simulink model "question3Sim"  (R2014a)
settings: Solver=ode45  StartTime=0.0  StopTime=2  RelTol=1e-3
settings Model: Creator=cunnia3  LastModifiedBy=cunnia3

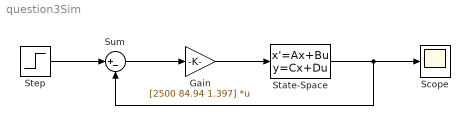
== system question3Sim ==
  Gain : Gain  Gain=[2500 84.94 1.397]  Multiplication=Matrix(K*u) (u vector)
  Scope : Scope
  State-Space : StateSpace  A=[0 1 0; 0 0 1; 0 -6 -20.3]  B=[0;0;100]  C=[1 0 0;0 1 0; 0 0 1]  D=[0; 0; 0]  X0=0
  Step : Step  After=[.01; 0; 0]  SampleTime=0
  Sum : Sum  Inputs=|+-
  wires:
  Step/1 -> Sum/1
  Sum/1 -> Gain/1
  Gain/1 -> State-Space/1
  State-Space/1 -> Sum/2, Scope/1
